simulink model "NDT_Localization"  (R2022a)
settings: Solver=FixedStepAuto  StartTime=0.0  StopTime=10.0  RelTol=1e-3
model workspace (MAT data in the model file):
  SL_ROS_VariableLengthArrays_MaxSizes : object (value not decoded)
undefined symbols (not defined in the file or in its folder): null
libraries: ros2lib x9, robotlib x8, simulink x1
(part 4 of 12)

== system NDT_Localization/observation_callback/check_localizer/If Action Subsystem/register_measurement_impl/If Action Subsystem/If Action Subsystem/solve/angle_params/If Action Subsystem3 ==
  y : Inport
  Action Port : ActionPort  ActionPortLabel=else
  Trigonometric Function : Trigonometry  Operator=cos
  Trigonometric Function1 : Trigonometry
  Out1 : Outport
  Out2 : Outport  Port=2
  wires:
  Trigonometric Function/1 -> Out1/1
  Trigonometric Function1/1 -> Out2/1
  y/1 -> Trigonometric Function1/1, Trigonometric Function/1

== system NDT_Localization/observation_callback/check_localizer/If Action Subsystem/register_measurement_impl/If Action Subsystem/If Action Subsystem/solve/angle_params/If Action Subsystem4 ==
  Action Port : ActionPort  ActionPortLabel=if(u1 > u2)
  Constant : Constant
  Constant1 : Constant  Value=0
  Out1 : Outport
  Out2 : Outport  Port=2
  wires:
  Constant/1 -> Out1/1
  Constant1/1 -> Out2/1

== system NDT_Localization/observation_callback/check_localizer/If Action Subsystem/register_measurement_impl/If Action Subsystem/If Action Subsystem/solve/angle_params/If Action Subsystem5 ==
  z : Inport
  Action Port : ActionPort  ActionPortLabel=else
  Trigonometric Function : Trigonometry  Operator=cos
  Trigonometric Function1 : Trigonometry
  Out1 : Outport
  Out2 : Outport  Port=2
  wires:
  Trigonometric Function1/1 -> Out2/1
  Trigonometric Function/1 -> Out1/1
  z/1 -> Trigonometric Function1/1, Trigonometric Function/1

== system NDT_Localization/map_callback/check_localizer/set_map/set_map_impl/insert/insert_/validate_pcl_map/check_fields/check_fields_name/For Iterator Subsystem ==
  In1 : Inport
  fields : Inport  Port=2
  ASCII to String : ASCIIToString
  Bus Selector2 : BusSelector  OutputSignals=name,offset
  Delay : Delay  DelayLength=1
  Delay1 : Delay  DelayLength=1
  For Iterator : ForIterator  IterationSource=external
  MATLAB Function : MATLAB Function  TreatAsAtomicUnit=on
  Selector : Selector  InputPortWidth=16  IndexOptions=Starting index (port)  Indices=[1 3]  OutputSizes=1
  name : Outport
  offset : Outport  Port=2
  wires:
  In1/1 -> For Iterator/1
  Selector/1 -> Bus Selector2/1  "field"
  fields/1 -> Selector/1
  Bus Selector2/1 -> ASCII to String/1  "<name>"
  Delay/1 -> MATLAB Function/1("data ")
  MATLAB Function/1(data) -> Delay/1, name/1
  For Iterator/1 -> Selector/2, MATLAB Function/2(index)  "index"
  ASCII to String/1 -> MATLAB Function/3(name)
  Bus Selector2/2 -> MATLAB Function/4(offset)  "<offset>"
  MATLAB Function/2(data1) -> Delay1/1, offset/1
  Delay1/1 -> MATLAB Function/5("data1 ")

== system NDT_Localization/map_callback/check_localizer/set_map/set_map_impl/insert/insert_/validate_pcl_map/check_fields/check_fields_name/For Iterator Subsystem1 ==
  In2 : Inport
  name : Inport  Port=2
  names : Inport  Port=3
  msg : Inport  Port=4
  Data Type Conversion : DataTypeConversion  OutDataTypeStr=uint8  SaturateOnIntegerOverflow=off  RndMeth=Floor
  Delay : Delay  DelayLength=1
  For Iterator : ForIterator  IterationSource=external
  If : If  IfExpression=u1 == 0
  If Action Subsystem : Subsystem  TreatAsAtomicUnit=on
  If Action Subsystem1 : Subsystem  TreatAsAtomicUnit=on
  Logical Operator : Logic  AllPortsSameDT=off  OutDataTypeStr=boolean
  MATLAB Function : MATLAB Function  TreatAsAtomicUnit=on
  Merge : Merge
  String Compare : StringCompare
  Out1 : Outport
  ret : Outport  Port=2
  wires:
  name/1 -> MATLAB Function/2(name)
  In2/1 -> For Iterator/1
  For Iterator/1 -> MATLAB Function/1(index)
  names/1 -> MATLAB Function/3(data)
  MATLAB Function/1(name_o) -> String Compare/1
  MATLAB Function/2(fields) -> String Compare/2
  String Compare/1 -> Logical Operator/2
  Logical Operator/1 -> Data Type Conversion/1, Delay/1
  Delay/1 -> Logical Operator/1
  Data Type Conversion/1 -> If/1
  If Action Subsystem/1(Out1) -> Merge/1
  If/1 -> If Action Subsystem/Action
  If/2 -> If Action Subsystem1/Action
  If Action Subsystem1/1(Out1) -> Merge/2
  msg/1 -> If Action Subsystem1/1(msg)
  Merge/1 -> Out1/1
  If Action Subsystem1/2(ret) -> ret/1

== system NDT_Localization/observation_callback/check_localizer/If Action Subsystem/register_measurement_impl/If Action Subsystem/If Action Subsystem/solve/If Action Subsystem1/For Iterator Subsystem/For Iterator Subsystem ==
  data : Inport
  myu : Inport  Port=2
  sigma : Inport  Port=3
  outlier_ratio : Inport  Port=4
  voxel_size_x : Inport  Port=5
  voxel_size_y : Inport  Port=6
  voxel_size_z : Inport  Port=7
  set_jacobian : Inport  Port=8
  set_gradient : Inport  Port=9
  set_hessian : Inport  Port=10
  point_hessian : Inport  Port=11
  Affine : MATLAB Function  TreatAsAtomicUnit=on
  Delay : Delay  DelayLength=1
  For Iterator : ForIterator  IterationSource=external
  For Iterator Subsystem : Subsystem  TreatAsAtomicUnit=on
  MATLAB Function : MATLAB Function  TreatAsAtomicUnit=on
  Width : Width
  gradient_jaco : Subsystem
  make_c_param : Subsystem
  make_d_param : Subsystem
  score : Subsystem
  score_out : Outport
  jacobian_out : Outport  Port=2
  hessian_out : Outport  Port=3
  wires:
  make_c_param/1(c1) -> make_d_param/1(c1)
  voxel_size_z/1 -> make_c_param/4(voxel_size_z)
  outlier_ratio/1 -> make_c_param/1(outlier_ratio)
  make_d_param/2(d2) -> For Iterator Subsystem/9(d2), gradient_jaco/9(d2), score/6(d2)
  voxel_size_y/1 -> make_c_param/3(voxel_size_y)
  make_c_param/2(c2) -> make_d_param/2(c2)
  voxel_size_x/1 -> make_c_param/2(voxel_size_x)
  make_d_param/1(d1) -> For Iterator Subsystem/8(d1), score/5(d1), gradient_jaco/8(d1)
  Width/1 -> For Iterator/1
  For Iterator/1 -> For Iterator Subsystem/3(i), gradient_jaco/3(index), MATLAB Function/2(index)
  MATLAB Function/1(pt) -> Affine/1(u)
  Affine/1(out) -> score/4(x), For Iterator Subsystem/4(data), gradient_jaco/4(data)
  sigma/1 -> For Iterator Subsystem/5(sigma), score/2(sigma), gradient_jaco/5(sigma)
  myu/1 -> gradient_jaco/6(myu), For Iterator Subsystem/6(myu), score/3(myu)
  score/1(p) -> score_out/1, Delay/1
  Delay/1 -> score/1(score)
  set_jacobian/1 -> gradient_jaco/1(set_jacobian)
  gradient_jaco/1(Out1) -> jacobian_out/1
  set_gradient/1 -> For Iterator Subsystem/2(set_gradient), gradient_jaco/2(set_gradient)
  set_hessian/1 -> For Iterator Subsystem/1(set_hessian)
  data/1 -> For Iterator Subsystem/7(x), gradient_jaco/7(x), MATLAB Function/1(data), Width/1
  point_hessian/1 -> For Iterator Subsystem/10(point_hessian)
  For Iterator Subsystem/1(Out1) -> hessian_out/1

== system NDT_Localization/observation_callback/check_localizer/If Action Subsystem/register_measurement_impl/If Action Subsystem/If Action Subsystem/solve/If Action Subsystem1/For Iterator Subsystem/If Action Subsystem ==
  opt_direction.norm : Inport
  nr_iterations : Inport  Port=2
  Action Port : ActionPort  ActionPortLabel=if(u1 == 0 & u2 == 0 & u3 == 0 & u4 == 0)
  Bus Creator : BusCreator  Inputs=3
  termination_type.FAILURE : Constant  Value=2  OutDataTypeStr=uint32
  Out1 : Outport
  wires:
  Bus Creator/1 -> Out1/1  "OptimizationSummary"
  termination_type.FAILURE/1 -> Bus Creator/2  "termination_type"
  nr_iterations/1 -> Bus Creator/3
  opt_direction.norm/1 -> Bus Creator/1

== system NDT_Localization/observation_callback/check_localizer/If Action Subsystem/register_measurement_impl/If Action Subsystem/If Action Subsystem/solve/If Action Subsystem1/For Iterator Subsystem/If Action Subsystem1 ==
  opt_direction.norm : Inport
  nr_iterations : Inport  Port=2
  Action Port : ActionPort  ActionPortLabel=elseif(u5 <= u6)
  Bus Creator : BusCreator  Inputs=3
  termination_type.CONVERGENCE : Constant  OutDataTypeStr=uint32
  Out1 : Outport
  wires:
  termination_type.CONVERGENCE/1 -> Bus Creator/2  "termination_type"
  Bus Creator/1 -> Out1/1  "OptimizationSummary"
  nr_iterations/1 -> Bus Creator/3
  opt_direction.norm/1 -> Bus Creator/1

== system NDT_Localization/observation_callback/check_localizer/If Action Subsystem/register_measurement_impl/If Action Subsystem/If Action Subsystem/solve/If Action Subsystem1/For Iterator Subsystem/If Action Subsystem2 ==
  opt_direction.norm : Inport
  nr_iterations : Inport  Port=2
  Action Port : ActionPort  ActionPortLabel=else
  Bus Creator : BusCreator  Inputs=3
  termination_type.FAILURE : Constant  Value=2  OutDataTypeStr=uint32
  Out1 : Outport
  wires:
  termination_type.FAILURE/1 -> Bus Creator/2  "termination_type"
  Bus Creator/1 -> Out1/1  "OptimizationSummary"
  nr_iterations/1 -> Bus Creator/3
  opt_direction.norm/1 -> Bus Creator/1

== system NDT_Localization/observation_callback/check_localizer/If Action Subsystem/register_measurement_impl/If Action Subsystem/If Action Subsystem/solve/If Action Subsystem1/For Iterator Subsystem/angle_params ==
  pose : Inport
  Bus Creator : BusCreator  Inputs=6
  If : If  NumInputs=2  IfExpression=u1 > u2
  If Action Subsystem : Subsystem  TreatAsAtomicUnit=on
  If Action Subsystem1 : Subsystem  TreatAsAtomicUnit=on
  If Action Subsystem2 : Subsystem  TreatAsAtomicUnit=on
  If Action Subsystem3 : Subsystem  TreatAsAtomicUnit=on
  If Action Subsystem4 : Subsystem  TreatAsAtomicUnit=on
  If Action Subsystem5 : Subsystem  TreatAsAtomicUnit=on
  If1 : If  NumInputs=2  IfExpression=u1 > u2
  If2 : If  NumInputs=2  IfExpression=u1 > u2
  MATLAB Function : MATLAB Function  TreatAsAtomicUnit=on
  Merge{,1..5} (6 alike) : Merge
  approx_thresh : Constant  Value=0.00010
  params : Outport
  wires:
  pose/1 -> MATLAB Function/1(u)
  MATLAB Function/1(x) -> If/2, If Action Subsystem1/1(x)
  MATLAB Function/3(z) -> If2/2, If Action Subsystem5/1(z)
  MATLAB Function/2(y) -> If Action Subsystem3/1(y), If1/2
  If Action Subsystem1/1(Out1) -> Merge/2
  If Action Subsystem1/2(Out2) -> Merge1/2
  If Action Subsystem3/1(Out1) -> Merge2/2
  If Action Subsystem3/2(Out2) -> Merge3/2
  If Action Subsystem5/1(Out1) -> Merge4/2
  If Action Subsystem5/2(Out2) -> Merge5/2
  approx_thresh/1 -> If2/1, If1/1, If/1
  If/1 -> If Action Subsystem/Action
  If/2 -> If Action Subsystem1/Action
  If1/1 -> If Action Subsystem2/Action
  If1/2 -> If Action Subsystem3/Action
  If2/2 -> If Action Subsystem5/Action
  If2/1 -> If Action Subsystem4/Action
  If Action Subsystem/1(Out1) -> Merge/1
  If Action Subsystem/2(Out2) -> Merge1/1
  If Action Subsystem2/1(Out1) -> Merge2/1
  If Action Subsystem2/2(Out2) -> Merge3/1
  If Action Subsystem4/1(Out1) -> Merge4/1
  If Action Subsystem4/2(Out2) -> Merge5/1
  Bus Creator/1 -> params/1
  Merge/1 -> Bus Creator/1  "cx"
  Merge1/1 -> Bus Creator/2  "sx"
  Merge2/1 -> Bus Creator/3  "cy"
  Merge3/1 -> Bus Creator/4  "sy"
  Merge4/1 -> Bus Creator/5  "cz"
  Merge5/1 -> Bus Creator/6  "sz"

== system NDT_Localization/observation_callback/check_localizer/If Action Subsystem/register_measurement_impl/If Action Subsystem/If Action Subsystem/solve/If Action Subsystem1/For Iterator Subsystem/compute_next_step ==
  eig_pose : Inport
  opt_direction : Inport  Port=2
  problem : Inport  Port=3
  localizer_ptr : Inport  Port=4
  Add4 : Sum  Inputs=+
  Bus Selector : BusSelector  OutputSignals=OptimizerT.MoreThuenteLineSearch.max_step,OptimizerT.MoreThuenteLineSearch.min_step
  If : If  NumInputs=2  IfExpression=u1 < u2
  If Action Subsystem : Subsystem  TreatAsAtomicUnit=on
  If Action Subsystem1 : Subsystem  TreatAsAtomicUnit=on
  Math Function2 : Math  Operator=square
  Merge : Merge
  Min : MinMax  Inputs=2
  step : Outport
  wires:
  Merge/1 -> step/1
  Math Function2/1 -> Add4/1
  opt_direction/1 -> If Action Subsystem1/3(opt_direction), If Action Subsystem/1(opt_direction), Math Function2/1
  localizer_ptr/1 -> If Action Subsystem1/5(localizer_ptr), Bus Selector/1
  Bus Selector/2 -> If/2  "<min_step>"
  Add4/1 -> Min/1  "step_norm"
  Bus Selector/1 -> Min/2  "<max_step>"
  Min/1 -> If Action Subsystem1/1(a_t), If/1  "a_t"
  If/2 -> If Action Subsystem1/Action
  If/1 -> If Action Subsystem/Action
  If Action Subsystem/1(Out1) -> Merge/1
  If Action Subsystem1/1(Out1) -> Merge/2
  eig_pose/1 -> If Action Subsystem1/2(eig_pose)
  problem/1 -> If Action Subsystem1/4(problem)

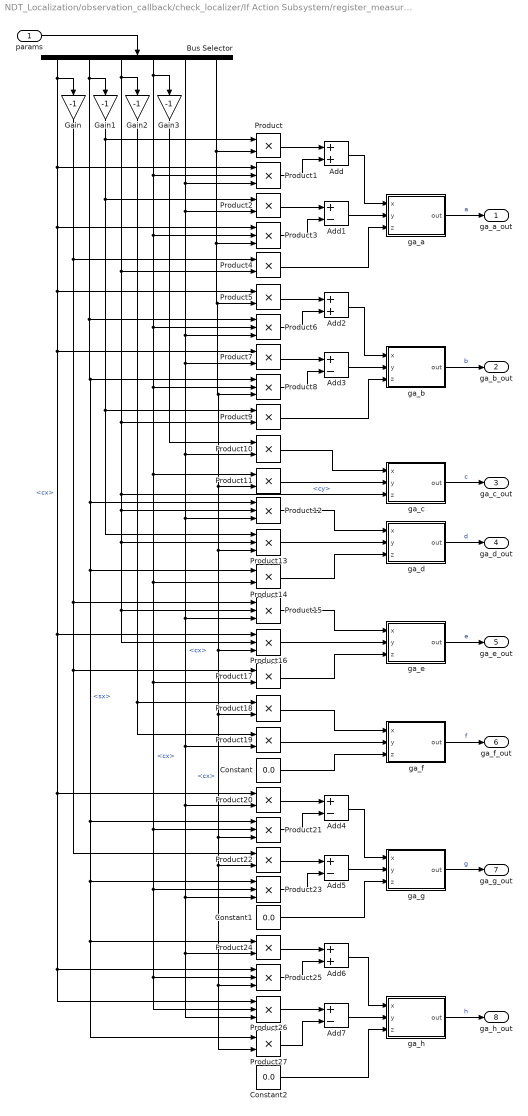
== system NDT_Localization/observation_callback/check_localizer/If Action Subsystem/register_measurement_impl/If Action Subsystem/If Action Subsystem/solve/If Action Subsystem1/For Iterator Subsystem/gradient_angle ==
  params : Inport
  Add : Sum
  Add{1,3..5,7} (5 alike) : Sum  Inputs=+-
  Add2 : Sum
  Add6 : Sum
  Bus Selector : BusSelector  OutputSignals=cx,sx,cy,sy,cz,sz
  Constant : Constant  Value=0.0
  Constant1 : Constant  Value=0.0
  Constant2 : Constant  Value=0.0
  Gain{,1..3} (4 alike) : Gain  Gain=-1
  Product{,2,4..5,7,9..11,14,17..20,22,24,27} (16 alike) : Product
  Product{1,3,6,8,12..13,15..16,21,23,25..26} (12 alike) : Product  Inputs=3
  ga_a : MATLAB Function  TreatAsAtomicUnit=on
  ga_b : MATLAB Function  TreatAsAtomicUnit=on
  ga_c : MATLAB Function  TreatAsAtomicUnit=on
  ga_d : MATLAB Function  TreatAsAtomicUnit=on
  ga_e : MATLAB Function  TreatAsAtomicUnit=on
  ga_f : MATLAB Function  TreatAsAtomicUnit=on
  ga_g : MATLAB Function  TreatAsAtomicUnit=on
  ga_h : MATLAB Function  TreatAsAtomicUnit=on
  ga_a_out : Outport
  ga_b_out : Outport  Port=2
  ga_c_out : Outport  Port=3
  ga_d_out : Outport  Port=4
  ga_e_out : Outport  Port=5
  ga_f_out : Outport  Port=6
  ga_g_out : Outport  Port=7
  ga_h_out : Outport  Port=8
  wires:
  params/1 -> Bus Selector/1
  Bus Selector/1 -> Product1/1, Product16/1, Product25/1, Product26/1, Product20/1, Product7/1, Product5/1, Product3/1, Gain/1  "<cx>"
  Bus Selector/2 -> Product6/1, Product12/1, Product14/1, Product21/1, Product23/1, Product27/1, Product24/1, Product8/1, Gain1/1  "<sx>"
  Bus Selector/3 -> Product12/2, Product13/2, Product15/2, Product16/2, ga_c/3(z), Product9/2, Product4/2, Gain2/1  "<cy>"
  Bus Selector/4 -> Product11/1, Product14/2, Product17/2, Product21/2, Product25/2, Product26/2, Product23/2, Product8/2, Product6/2, Product3/2, Product1/2, Gain3/1  "<cx>"
  Bus Selector/5 -> Product6/3, Product10/2, Product12/3, Product15/3, Product19/2, Product20/2, Product23/3, Product26/3, Product24/2, Product7/2, Product2/2, Product1/3  "<cx>"
  Bus Selector/6 -> Product11/2, Product13/3, Product16/3, Product18/2, Product21/3, Product22/2, Product25/3, Product27/2, Product8/3, Product5/2, Product3/3, Product/2  "<cx>"
  Gain1/1 -> Product13/1, Product9/1, Product2/1, Product/1
  Product/1 -> Add/1
  Product1/1 -> Add/2
  Product2/1 -> Add1/1
  Add/1 -> ga_a/1(x)
  Add1/1 -> ga_a/2(y)
  Gain/1 -> Product15/1, Product17/1, Product22/1, Product4/1
  Product4/1 -> ga_a/3(z)
  Product3/1 -> Add1/2
  Product6/1 -> Add2/2
  Product7/1 -> Add3/1
  Product8/1 -> Add3/2
  Product5/1 -> Add2/1
  Add2/1 -> ga_b/1(x)
  Product9/1 -> ga_b/3(z)
  Add3/1 -> ga_b/2(y)
  Product11/1 -> ga_c/2(y)
  Product10/1 -> ga_c/1(x)
  Gain2/1 -> Product18/1, Product19/1
  Gain3/1 -> Product10/1
  Product13/1 -> ga_d/2(y)
  Product12/1 -> ga_d/1(x)
  Product14/1 -> ga_d/3(z)
  Product19/1 -> ga_f/2(y)
  Constant/1 -> ga_f/3(z)
  Product18/1 -> ga_f/1(x)
  Product16/1 -> ga_e/2(y)
  Product17/1 -> ga_e/3(z)
  Product15/1 -> ga_e/1(x)
  Product21/1 -> Add4/2
  Product22/1 -> Add5/1
  Product23/1 -> Add5/2
  Product20/1 -> Add4/1
  Add5/1 -> ga_g/2(y)
  Product25/1 -> Add6/2
  Product26/1 -> Add7/1
  Product27/1 -> Add7/2
  Product24/1 -> Add6/1
  Constant1/1 -> ga_g/3(z)
  Add4/1 -> ga_g/1(x)
  Add7/1 -> ga_h/2(y)
  Add6/1 -> ga_h/1(x)
  Constant2/1 -> ga_h/3(z)
  ga_a/1(out) -> ga_a_out/1  "a"
  ga_b/1(out) -> ga_b_out/1  "b"
  ga_c/1(out) -> ga_c_out/1  "c"
  ga_d/1(out) -> ga_d_out/1  "d"
  ga_e/1(out) -> ga_e_out/1  "e"
  ga_f/1(out) -> ga_f_out/1  "f"
  ga_g/1(out) -> ga_g_out/1  "g"
  ga_h/1(out) -> ga_h_out/1  "h"

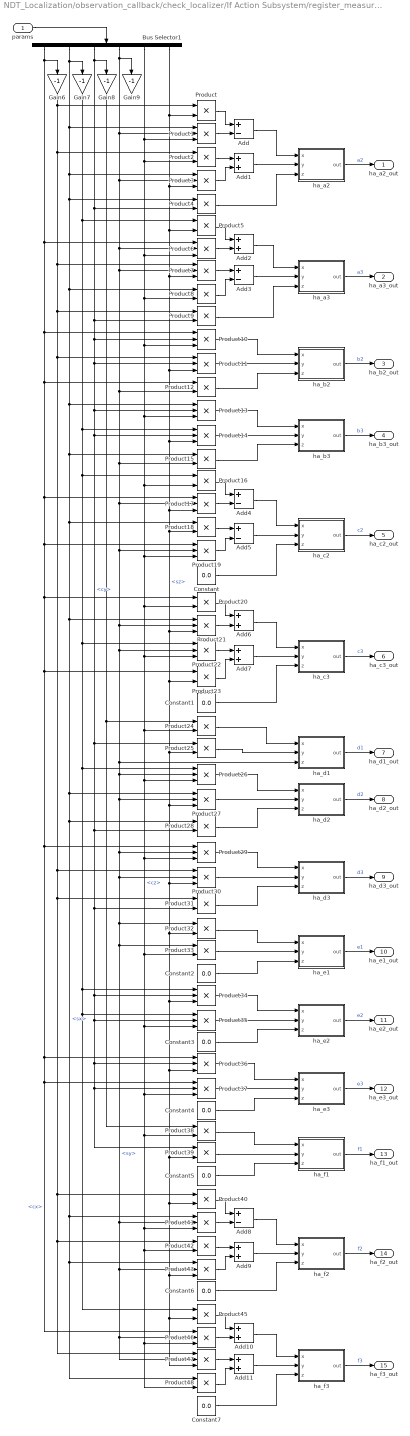
== system NDT_Localization/observation_callback/check_localizer/If Action Subsystem/register_measurement_impl/If Action Subsystem/If Action Subsystem/solve/If Action Subsystem1/For Iterator Subsystem/hessian_angle ==
  params : Inport
  Add{,3..5,8} (5 alike) : Sum  Inputs=+-
  Add{1..2,6..7,9..11} (7 alike) : Sum
  Bus Selector1 : BusSelector  OutputSignals=cx,sx,cy,sy,cz,sz
  Constant{,1..7} (8 alike) : Constant  Value=0.0
  Gain{6..9} (4 alike) : Gain  Gain=-1
  Product{,2,4..5,8..9,12,15..16,18,20,23..25,28,31..33,38..40,42,45,48} (24 alike) : Product
  Product{1,3,6..7,10..11,13..14,17,19,21..22,26..27,29..30,34..37,41,43,46..47} (24 alike) : Product  Inputs=3
  ha_a2 : MATLAB Function  TreatAsAtomicUnit=on
  ha_a3 : MATLAB Function  TreatAsAtomicUnit=on
  ha_b2 : MATLAB Function  TreatAsAtomicUnit=on
  ha_b3 : MATLAB Function  TreatAsAtomicUnit=on
  ha_c2 : MATLAB Function  TreatAsAtomicUnit=on
  ha_c3 : MATLAB Function  TreatAsAtomicUnit=on
  ha_d1 : MATLAB Function  TreatAsAtomicUnit=on
  ha_d2 : MATLAB Function  TreatAsAtomicUnit=on
  ha_d3 : MATLAB Function  TreatAsAtomicUnit=on
  ha_e1 : MATLAB Function  TreatAsAtomicUnit=on
  ha_e2 : MATLAB Function  TreatAsAtomicUnit=on
  ha_e3 : MATLAB Function  TreatAsAtomicUnit=on
  ha_f1 : MATLAB Function  TreatAsAtomicUnit=on
  ha_f2 : MATLAB Function  TreatAsAtomicUnit=on
  ha_f3 : MATLAB Function  TreatAsAtomicUnit=on
  ha_a2_out : Outport
  ha_a3_out : Outport  Port=2
  ha_b2_out : Outport  Port=3
  ha_b3_out : Outport  Port=4
  ha_c2_out : Outport  Port=5
  ha_c3_out : Outport  Port=6
  ha_d1_out : Outport  Port=7
  ha_d2_out : Outport  Port=8
  ha_d3_out : Outport  Port=9
  ha_e1_out : Outport  Port=10
  ha_e2_out : Outport  Port=11
  ha_e3_out : Outport  Port=12
  ha_f1_out : Outport  Port=13
  ha_f2_out : Outport  Port=14
  ha_f3_out : Outport  Port=15
  wires:
  Bus Selector1/1 -> Product6/1, Product10/1, Product12/1, Product17/1, Product19/1, Product20/1, Product23/1, Product29/1, Product36/1, Product37/1, Product46/1, Gain6/1  "<cx>"
  Bus Selector1/3 -> Product4/2, Product9/2, Product10/2, Product11/2, Product13/2, Product14/2, Product25/1, Product28/2, Product31/2, Product34/2, Product35/2, Product36/2, Product37/2, Product39/1, Gain8/1  "<cy>"
  Bus Selector1/4 -> Product1/2, Product3/2, Product6/2, Product7/2, Product15/2, Product17/2, Product19/2, ha_d1/3(z), Product27/2, Product29/2, Product30/2, Product32/1, Product33/1, Product41/2, Product43/2, Product47/2, Product46/2, Product26/2, Product22/2, Product21/2, Product12/2, Gain9/1  "<sy>"
  params/1 -> Bus Selector1/1
  Bus Selector1/2 -> Product1/1, Product3/1, Product4/1, Product8/1, Product13/1, Product15/1, Product18/1, Product21/1, Product27/1, Product28/1, Product41/1, Product43/1, Product48/1, Gain7/1  "<sx>"
  Bus Selector1/5 -> Product1/3, Product2/2, Product6/3, Product8/2, Product10/3, Product13/3, Product16/2, Product19/3, Product20/2, Product22/3, Product24/2, Product26/3, Product29/3, Product33/2, Product35/3, Product37/3, Product38/2, Product41/3, Product42/2, Product46/3, Product48/2  "<cz>"
  Bus Selector1/6 -> Product/2, Product3/3, Product5/2, Product7/3, Product11/3, Product14/3, Product17/3, Product18/2, Product21/3, Product23/2, Product25/2, Product30/3, Product32/2, Product34/3, Product36/3, Product39/2, Product40/2, Product43/3, Product45/2, Product47/3, Product27/3  "<sz>"
  ha_a2/1(out) -> ha_a2_out/1  "a2"
  ha_a3/1(out) -> ha_a3_out/1  "a3"
  ha_b3/1(out) -> ha_b3_out/1  "b3"
  ha_b2/1(out) -> ha_b2_out/1  "b2"
  ha_c3/1(out) -> ha_c3_out/1  "c3"
  ha_c2/1(out) -> ha_c2_out/1  "c2"
  ha_d3/1(out) -> ha_d3_out/1  "d3"
  ha_d2/1(out) -> ha_d2_out/1  "d2"
  ha_d1/1(out) -> ha_d1_out/1  "d1"
  ha_e1/1(out) -> ha_e1_out/1  "e1"
  ha_e3/1(out) -> ha_e3_out/1  "e3"
  ha_e2/1(out) -> ha_e2_out/1  "e2"
  ha_f1/1(out) -> ha_f1_out/1  "f1"
  ha_f3/1(out) -> ha_f3_out/1  "f3"
  ha_f2/1(out) -> ha_f2_out/1  "f2"
  Product1/1 -> Add/2
  Product/1 -> Add/1
  Product2/1 -> Add1/1
  Product3/1 -> Add1/2
  Product4/1 -> ha_a2/3(z)
  Add1/1 -> ha_a2/2(y)
  Add/1 -> ha_a2/1(x)
  Product9/1 -> ha_a3/3(z)
  Add3/1 -> ha_a3/2(y)
  Product8/1 -> Add3/2
  Product7/1 -> Add3/1
  Product6/1 -> Add2/2
  Product5/1 -> Add2/1
  Add2/1 -> ha_a3/1(x)
  Product11/1 -> ha_b2/2(y)
  Product10/1 -> ha_b2/1(x)
  Product12/1 -> ha_b2/3(z)
  Product14/1 -> ha_b3/2(y)
  Product13/1 -> ha_b3/1(x)
  Product15/1 -> ha_b3/3(z)
  Product19/1 -> Add5/2
  Product18/1 -> Add5/1
  Product17/1 -> Add4/2
  Product16/1 -> Add4/1
  Product23/1 -> Add7/2
  Product22/1 -> Add7/1
  Product21/1 -> Add6/2
  Product20/1 -> Add6/1
  Add5/1 -> ha_c2/2(y)
  Constant/1 -> ha_c2/3(z)
  Add4/1 -> ha_c2/1(x)
  Add7/1 -> ha_c3/2(y)
  Constant1/1 -> ha_c3/3(z)
  Add6/1 -> ha_c3/1(x)
  Product25/1 -> ha_d1/2(y)
  Product24/1 -> ha_d1/1(x)
  Product27/1 -> ha_d2/2(y)
  Product28/1 -> ha_d2/3(z)
  Product26/1 -> ha_d2/1(x)
  Product30/1 -> ha_d3/2(y)
  Product29/1 -> ha_d3/1(x)
  Product31/1 -> ha_d3/3(z)
  Product33/1 -> ha_e1/2(y)
  Product32/1 -> ha_e1/1(x)
  Constant2/1 -> ha_e1/3(z)
  Product35/1 -> ha_e2/2(y)
  Product34/1 -> ha_e2/1(x)
  Constant3/1 -> ha_e2/3(z)
  Constant4/1 -> ha_e3/3(z)
  Product37/1 -> ha_e3/2(y)
  Product36/1 -> ha_e3/1(x)
  Constant5/1 -> ha_f1/3(z)
  Product38/1 -> ha_f1/1(x)
  Product39/1 -> ha_f1/2(y)
  Product42/1 -> Add9/1
  Product41/1 -> Add8/2
  Product46/1 -> Add10/2
  Product48/1 -> Add11/2
  Product43/1 -> Add9/2
  Product40/1 -> Add8/1
  Product47/1 -> Add11/1
  Product45/1 -> Add10/1
  Add9/1 -> ha_f2/2(y)
  Add11/1 -> ha_f3/2(y)
  Add10/1 -> ha_f3/1(x)
  Add8/1 -> ha_f2/1(x)
  Constant6/1 -> ha_f2/3(z)
  Constant7/1 -> ha_f3/3(z)
  Gain7/1 -> Product5/1, Product14/1, Product16/1, Product22/1, Product34/1, Product35/1, Product45/1, Product26/1
  Gain8/1 -> Product24/1, Product38/1
  Gain6/1 -> Product2/1, Product7/1, Product9/1, Product11/1, Product30/1, Product31/1, Product40/1, Product42/1, Product47/1, Product/1

== system NDT_Localization/map_callback/check_localizer/set_map/set_map_impl/insert/insert_/validate_pcl_map/check_fields/check_fields_name/For Iterator Subsystem1/If Action Subsystem ==
  Action Port : ActionPort  ActionPortLabel=if(u1 == 0)
  Constant : Constant  Value=0
  Out1 : Outport
  wires:
  Constant/1 -> Out1/1

== system NDT_Localization/map_callback/check_localizer/set_map/set_map_impl/insert/insert_/validate_pcl_map/check_fields/check_fields_name/For Iterator Subsystem1/If Action Subsystem1 ==
  msg : Inport
  Action Port : ActionPort  ActionPortLabel=else
  Add : Sum  Inputs=+-
  Bus Selector : BusSelector  OutputSignals=data,row_step,width,point_step
  Constant : Constant
  Divide : Product  Inputs=*/
  Math Function : Math  Operator=mod
  Min : MinMax  Inputs=3
  Product : Product
  Width : Width
  Out1 : Outport
  ret : Outport  Port=2
  wires:
  msg/1 -> Bus Selector/1
  Constant/1 -> Out1/1
  Bus Selector/1 -> Width/1  "<data>"
  Width/1 -> Min/1
  Product/1 -> Min/3
  Bus Selector/4 -> Math Function/2, Divide/2, Product/2  "<point_step>"
  Bus Selector/2 -> Min/2  "<row_step>"
  Bus Selector/3 -> Product/1  "<width>"
  Min/1 -> Add/1, Math Function/1  "min_data_length"
  Math Function/1 -> Add/2
  Add/1 -> Divide/1  "safe_data_length"
  Divide/1 -> ret/1

== system NDT_Localization/observation_callback/check_localizer/If Action Subsystem/register_measurement_impl/If Action Subsystem/If Action Subsystem/solve/If Action Subsystem1/For Iterator Subsystem/For Iterator Subsystem/For Iterator Subsystem ==
  set_hessian : Inport
  set_gradient : Inport  Port=2
  i : Inport  Port=3
  data : Inport  Port=4
  sigma : Inport  Port=5
  myu : Inport  Port=6
  x : Inport  Port=7
  d1 : Inport  Port=8
  d2 : Inport  Port=9
  point_hessian : Inport  Port=10
  Add : Sum  Inputs=+-
  Add1 : Sum  Inputs=+++
  Constant : Constant  Value=-2
  Divide1 : Product  Inputs=*/
  For Iterator : ForIterator  IterationSource=external
  MATLAB Function : MATLAB Function  TreatAsAtomicUnit=on
  MATLAB Function1 : MATLAB Function  TreatAsAtomicUnit=on
  Math Function : Math
  Math Function1 : Math  Operator=transpose
  Math Function2 : Math  Operator=reciprocal
  Product : Product  Inputs=4
  Product1 : Product  Inputs=3  Multiplication=Matrix(*)
  Product{4,6,8,10} (4 alike) : Product  Multiplication=Matrix(*)
  Product{2..3,5,7,9} (5 alike) : Product
  gradient_col_i : MATLAB Function  TreatAsAtomicUnit=on
  gradient_col_j : MATLAB Function  TreatAsAtomicUnit=on
  hessian_add : MATLAB Function  TreatAsAtomicUnit=on
  Out1 : Outport
  wires:
  Product3/1 -> Product8/2, Product4/2
  Product4/1 -> Product7/1
  Constant/1 -> Divide1/2
  set_gradient/1 -> gradient_col_j/2(gradient), gradient_col_i/2(gradient)
  hessian_add/1(hessian) -> Out1/1
  set_hessian/1 -> MATLAB Function/1(u), hessian_add/1("hessian ")
  i/1 -> hessian_add/2(index_i), gradient_col_i/1(index_i), MATLAB Function1/1(index_i)
  sigma/1 -> Math Function2/1
  Product/1 -> hessian_add/4(num)
  gradient_col_i/1(y) -> Product3/2
  data/1 -> Product10/1, Product6/1, Product4/1
  Add/1 -> Product1/3, Math Function1/1  "x-myu"
  d2/1 -> Divide1/1, Product/3  "d2"
  Product2/1 -> Math Function/1
  Divide1/1 -> Product2/1
  Math Function/1 -> Product/4
  Math Function1/1 -> Product1/1
  x/1 -> Add/1
  d1/1 -> Product/2  "d1"
  Product1/1 -> Product2/2
  myu/1 -> Add/2
  Math Function2/1 -> Product5/1, Product3/1, Product9/1, Product1/2  "inv_cov"
  MATLAB Function/1(y) -> For Iterator/1
  For Iterator/1 -> hessian_add/3(index_j), MATLAB Function1/2(index_j), gradient_col_j/1(index_j)
  Product5/1 -> Product6/2
  gradient_col_j/1(y) -> Product8/1, Product5/2
  Product6/1 -> Product7/2
  Product7/1 -> Add1/1
  Add1/1 -> Product/1
  Product8/1 -> Add1/3
  Product9/1 -> Product10/2
  Product10/1 -> Add1/2
  point_hessian/1 -> MATLAB Function1/3(point_hessian)
  MATLAB Function1/1(y) -> Product9/2

== system NDT_Localization/observation_callback/check_localizer/If Action Subsystem/register_measurement_impl/If Action Subsystem/If Action Subsystem/solve/If Action Subsystem1/For Iterator Subsystem/For Iterator Subsystem/gradient_jaco ==
  set_jacobian : Inport
  set_gradient : Inport  Port=2
  index : Inport  Port=3
  data : Inport  Port=4
  sigma : Inport  Port=5
  myu : Inport  Port=6
  x : Inport  Port=7
  d1 : Inport  Port=8
  d2 : Inport  Port=9
  Add : Sum  Inputs=+-
  Constant : Constant  Value=-2
  Divide1 : Product  Inputs=*/
  Math Function : Math
  Math Function1 : Math  Operator=transpose
  Math Function2 : Math  Operator=reciprocal
  Product : Product  Inputs=4
  Product1 : Product  Inputs=3  Multiplication=Matrix(*)
  Product2 : Product
  Product3 : Product
  Product4 : Product  Multiplication=Matrix(*)
  gradient_col : MATLAB Function  TreatAsAtomicUnit=on
  jaco_add : MATLAB Function  TreatAsAtomicUnit=on
  Out1 : Outport
  wires:
  myu/1 -> Add/2
  Constant/1 -> Divide1/2
  Math Function1/1 -> Product1/1
  Divide1/1 -> Product2/1
  d2/1 -> Divide1/1, Product/3  "d2"
  Math Function2/1 -> Product3/2, Product1/2  "inv_cov"
  Product1/1 -> Product2/2
  d1/1 -> Product/2  "d1"
  x/1 -> Add/1
  Math Function/1 -> Product/4
  Product2/1 -> Math Function/1
  Add/1 -> Product1/3, Math Function1/1  "x-myu"
  sigma/1 -> Math Function2/1
  Product/1 -> jaco_add/3(num)
  index/1 -> jaco_add/2(index), gradient_col/1(index)
  jaco_add/1(jacobian) -> Out1/1
  set_jacobian/1 -> jaco_add/1("jacobian ")
  set_gradient/1 -> gradient_col/2(gradient)
  gradient_col/1(y) -> Product3/1
  data/1 -> Product4/1
  Product3/1 -> Product4/2
  Product4/1 -> Product/1

== system NDT_Localization/observation_callback/check_localizer/If Action Subsystem/register_measurement_impl/If Action Subsystem/If Action Subsystem/solve/If Action Subsystem1/For Iterator Subsystem/For Iterator Subsystem/make_c_param ==
  outlier_ratio : Inport
  voxel_size_x : Inport  Port=2
  voxel_size_y : Inport  Port=3
  voxel_size_z : Inport  Port=4
  Constant : Constant
  Divide : Product  Inputs=*/
  Gain : Gain  Gain=10
  Product : Product  Inputs=3
  Subtract : Sum  Inputs=+-
  c1 : Outport
  c2 : Outport  Port=2
  wires:
  Constant/1 -> Subtract/1
  outlier_ratio/1 -> Divide/1, Subtract/2
  Subtract/1 -> Gain/1
  Gain/1 -> c1/1
  Product/1 -> Divide/2
  Divide/1 -> c2/1
  voxel_size_y/1 -> Product/2
  voxel_size_z/1 -> Product/3
  voxel_size_x/1 -> Product/1

== system NDT_Localization/observation_callback/check_localizer/If Action Subsystem/register_measurement_impl/If Action Subsystem/If Action Subsystem/solve/If Action Subsystem1/For Iterator Subsystem/For Iterator Subsystem/make_d_param ==
  c1 : Inport
  c2 : Inport  Port=2
  Add1 : Sum
  Add2 : Sum  Inputs=-+
  Add3 : Sum
  Add4 : Sum  Inputs=+-
  Constant : Constant  Value=-2
  Constant1 : Constant  Value=-0.5
  Divide : Product  Inputs=*/
  Math Function{3..4,6..7} (4 alike) : Math  Operator=log
  Math Function5 : Math
  Product3 : Product
  Product4 : Product
  d1 : Outport
  d2 : Outport  Port=2
  wires:
  Add2/1 -> Divide/2, d1/1  "d1"
  Math Function4/1 -> Add4/1, Add2/2  "-d3"
  Product4/1 -> Add3/1
  Add3/1 -> Math Function6/1
  c1/1 -> Product4/1, Add1/1
  Constant/1 -> Product3/2
  Constant1/1 -> Math Function5/1
  Product3/1 -> d2/1  "d2"
  Math Function5/1 -> Product4/2
  Math Function7/1 -> Product3/1
  Divide/1 -> Math Function7/1
  Math Function6/1 -> Add4/2
  c2/1 -> Add3/2, Math Function4/1, Add1/2
  Add4/1 -> Divide/1
  Add1/1 -> Math Function3/1
  Math Function3/1 -> Add2/1

== system NDT_Localization/observation_callback/check_localizer/If Action Subsystem/register_measurement_impl/If Action Subsystem/If Action Subsystem/solve/If Action Subsystem1/For Iterator Subsystem/For Iterator Subsystem/score ==
  score : Inport
  sigma : Inport  Port=2
  myu : Inport  Port=3
  x : Inport  Port=4
  d1 : Inport  Port=5
  d2 : Inport  Port=6
  Add : Sum  Inputs=+-
  Add1 : Sum
  Constant : Constant  Value=-2
  Divide1 : Product  Inputs=*/
  Gain : Gain  Gain=-1
  Math Function : Math
  Math Function1 : Math  Operator=transpose
  Math Function2 : Math  Operator=reciprocal
  Product : Product
  Product1 : Product  Inputs=3  Multiplication=Matrix(*)
  Product2 : Product
  p : Outport
  wires:
  sigma/1 -> Math Function2/1
  Math Function/1 -> Product/2
  Gain/1 -> Product/1  "-d1"
  myu/1 -> Add/2
  x/1 -> Add/1
  Product2/1 -> Math Function/1
  Add/1 -> Product1/3, Math Function1/1  "x-myu"
  Product/1 -> Add1/2
  Math Function1/1 -> Product1/1
  Product1/1 -> Product2/2
  Math Function2/1 -> Product1/2
  Constant/1 -> Divide1/2
  Divide1/1 -> Product2/1
  d2/1 -> Divide1/1  "d2"
  d1/1 -> Gain/1
  Add1/1 -> p/1
  score/1 -> Add1/1

== system NDT_Localization/observation_callback/check_localizer/If Action Subsystem/register_measurement_impl/If Action Subsystem/If Action Subsystem/solve/If Action Subsystem1/For Iterator Subsystem/angle_params/If Action Subsystem ==
  Action Port : ActionPort
  Constant : Constant
  Constant1 : Constant  Value=0
  Out1 : Outport
  Out2 : Outport  Port=2
  wires:
  Constant/1 -> Out1/1
  Constant1/1 -> Out2/1

== system NDT_Localization/observation_callback/check_localizer/If Action Subsystem/register_measurement_impl/If Action Subsystem/If Action Subsystem/solve/If Action Subsystem1/For Iterator Subsystem/angle_params/If Action Subsystem1 ==
  x : Inport
  Action Port : ActionPort
  Trigonometric Function : Trigonometry  Operator=cos
  Trigonometric Function1 : Trigonometry
  Out1 : Outport
  Out2 : Outport  Port=2
  wires:
  x/1 -> Trigonometric Function1/1, Trigonometric Function/1
  Trigonometric Function1/1 -> Out2/1
  Trigonometric Function/1 -> Out1/1

== system NDT_Localization/observation_callback/check_localizer/If Action Subsystem/register_measurement_impl/If Action Subsystem/If Action Subsystem/solve/If Action Subsystem1/For Iterator Subsystem/angle_params/If Action Subsystem2 ==
  Action Port : ActionPort
  Constant : Constant
  Constant1 : Constant  Value=0
  Out1 : Outport
  Out2 : Outport  Port=2
  wires:
  Constant/1 -> Out1/1
  Constant1/1 -> Out2/1

== system NDT_Localization/observation_callback/check_localizer/If Action Subsystem/register_measurement_impl/If Action Subsystem/If Action Subsystem/solve/If Action Subsystem1/For Iterator Subsystem/angle_params/If Action Subsystem3 ==
  y : Inport
  Action Port : ActionPort
  Trigonometric Function : Trigonometry  Operator=cos
  Trigonometric Function1 : Trigonometry
  Out1 : Outport
  Out2 : Outport  Port=2
  wires:
  Trigonometric Function/1 -> Out1/1
  Trigonometric Function1/1 -> Out2/1
  y/1 -> Trigonometric Function1/1, Trigonometric Function/1

== system NDT_Localization/observation_callback/check_localizer/If Action Subsystem/register_measurement_impl/If Action Subsystem/If Action Subsystem/solve/If Action Subsystem1/For Iterator Subsystem/angle_params/If Action Subsystem4 ==
  Action Port : ActionPort
  Constant : Constant
  Constant1 : Constant  Value=0
  Out1 : Outport
  Out2 : Outport  Port=2
  wires:
  Constant/1 -> Out1/1
  Constant1/1 -> Out2/1

== system NDT_Localization/observation_callback/check_localizer/If Action Subsystem/register_measurement_impl/If Action Subsystem/If Action Subsystem/solve/If Action Subsystem1/For Iterator Subsystem/angle_params/If Action Subsystem5 ==
  z : Inport
  Action Port : ActionPort
  Trigonometric Function : Trigonometry  Operator=cos
  Trigonometric Function1 : Trigonometry
  Out1 : Outport
  Out2 : Outport  Port=2
  wires:
  Trigonometric Function1/1 -> Out2/1
  Trigonometric Function/1 -> Out1/1
  z/1 -> Trigonometric Function1/1, Trigonometric Function/1

== system NDT_Localization/observation_callback/check_localizer/If Action Subsystem/register_measurement_impl/If Action Subsystem/If Action Subsystem/solve/If Action Subsystem1/For Iterator Subsystem/compute_next_step/If Action Subsystem ==
  opt_direction : Inport
  Action Port : ActionPort  ActionPortLabel=if(u1 < u2)
  Out1 : Outport
  wires:
  opt_direction/1 -> Out1/1

== system NDT_Localization/observation_callback/check_localizer/If Action Subsystem/register_measurement_impl/If Action Subsystem/If Action Subsystem/solve/If Action Subsystem1/For Iterator Subsystem/compute_next_step/If Action Subsystem1 ==
  a_t : Inport
  eig_pose : Inport  Port=2
  opt_direction : Inport  Port=3
  problem : Inport  Port=4
  localizer_ptr : Inport  Port=5
  Action Port : ActionPort  ActionPortLabel=else
  Bus Creator : BusCreator  Inputs=4
  Bus Creator1 : BusCreator  Inputs=2
  Bus Creator2 : BusCreator  Inputs=2
  Bus Selector : BusSelector  OutputSignals=OptimizerT.MoreThuenteLineSearch.optimization_direction,OptimizerT.MoreThuenteLineSearch.mu,OptimizerT.MoreThuenteLineSearch.min_step,OptimizerT.MoreThuenteLineSearch.max_step,OptimizerT.MoreThuenteLineSearch.max_iterations
  Bus Selector1 : BusSelector  OutputSignals=min_step,max_step
  Constant : Constant  Value=0.0
  For Iterator Subsystem : Subsystem  TreatAsAtomicUnit=on
  If : If  NumInputs=2  IfExpression=u1 >= u2  ShowElse=off
  f_l : Subsystem
  f_u : Subsystem
  phi_0 : Subsystem
  phi_t : Subsystem  TreatAsAtomicUnit=on
  psi_t : Subsystem
  Out1 : Outport
  wires:
  Bus Selector/2 -> Bus Creator1/2  "<mu>"
  Bus Selector/1 -> Bus Creator/4  "<optimization_direction>"
  eig_pose/1 -> Bus Creator/1  "eig_pose"
  opt_direction/1 -> Bus Creator/2  "opt_direction"
  problem/1 -> Bus Creator/3  "problem"
  Bus Selector/3 -> Bus Creator2/1  "<min_step>"
  Bus Selector/4 -> Bus Creator2/2  "<max_step>"
  Bus Creator2/1 -> Bus Selector1/1  "interval"
  Bus Selector/5 -> For Iterator Subsystem/3(max_iterations)  "<max_iterations>"
  Bus Selector1/2 -> f_u/1(a_u)  "<max_step>"
  localizer_ptr/1 -> phi_0/3(localizer_ptr), For Iterator Subsystem/4(localizer_ptr), phi_t/3(localizer_ptr), psi_t/3(localizer_ptr), f_l/3(localizer_ptr), f_u/3(localizer_ptr), Bus Selector/1
  Bus Creator/1 -> For Iterator Subsystem/1(phi), phi_0/2(phi), phi_t/2(phi), Bus Creator1/1  "phi"
  If/1 -> phi_t/Action
  a_t/1 -> If/1, psi_t/1(a_t), phi_t/1(a_t)  "a_t"
  Bus Selector1/1 -> f_l/1(a_l)  "<min_step>"
  Constant/1 -> phi_0/1(step_size), If/2
  Bus Creator1/1 -> f_u/2(psi), f_l/2(psi), psi_t/2(psi), For Iterator Subsystem/2(psi)  "psi"
  phi_0/1(phi_0) -> For Iterator Subsystem/5(phi_0)
  phi_t/1(phi_t) -> For Iterator Subsystem/6(phi_t)
  psi_t/1(psi_t) -> For Iterator Subsystem/7(psi_t)
  f_l/1(f_l) -> For Iterator Subsystem/8(f_l)
  f_u/1(f_u) -> For Iterator Subsystem/9(f_u)
  For Iterator Subsystem/1(Out1) -> Out1/1

== system NDT_Localization/observation_callback/check_localizer/If Action Subsystem/register_measurement_impl/If Action Subsystem/If Action Subsystem/solve/If Action Subsystem1/For Iterator Subsystem/compute_next_step/If Action Subsystem1/For Iterator Subsystem ==
  phi : Inport
  psi : Inport  Port=2
  max_iterations : Inport  Port=3
  localizer_ptr : Inport  Port=4
  phi_0 : Inport  Port=5
  phi_t : Inport  Port=6
  psi_t : Inport  Port=7
  f_l : Inport  Port=8
  f_u : Inport  Port=9
  Abs : Abs  SaturateOnIntegerOverflow=off
  Abs1 : Abs  SaturateOnIntegerOverflow=off
  Add : Sum
  Add1 : Sum
  Bus Selector : BusSelector  OutputSignals=step_size,value,derivative
  Bus Selector1 : BusSelector  OutputSignals=step_size,value,derivative
  Bus Selector2 : BusSelector  OutputSignals=a_t,value,derivative
  Bus Selector5 : BusSelector  OutputSignals=OptimizerT.MoreThuenteLineSearch.eta
  Constant : Constant  Value=0.0
  Constant1 : Constant
  Constant2 : Constant
  Data Type Conversion : DataTypeConversion  OutDataTypeStr=uint8  SaturateOnIntegerOverflow=off  RndMeth=Floor
  Delay : Delay  DelayLength=1
  Delay1 : Delay  DelayLength=1  InitialCondition=true
  For Iterator : ForIterator  IterationSource=external  ExternalIncrement=on
  If : If  IfExpression=u1 == 0  ShowElse=off
  If Action Subsystem : Subsystem  TreatAsAtomicUnit=on
  Logical Operator : Logic  AllPortsSameDT=off  OutDataTypeStr=boolean
  Logical Operator1 : Logic  Operator=OR  AllPortsSameDT=off  OutDataTypeStr=boolean
  Product : Product
  Relational Operator : RelationalOperator  Operator=<=  OutDataTypeStr=boolean  RndMeth=Simplest  InputSameDT=off
  Relational Operator1 : RelationalOperator  OutDataTypeStr=boolean  RndMeth=Simplest  InputSameDT=off
  Switch : Switch  Criteria=u2 ~= 0  SaturateOnIntegerOverflow=off  InputSameDT=off
  Out1 : Outport
  wires:
  ? -> Out1/1
  max_iterations/1 -> Add1/1, For Iterator/1
  For Iterator/1 -> Delay/1  "step_iterations"
  phi_0/1 -> Bus Selector/1
  phi_t/1 -> If Action Subsystem/2(phi_t), Bus Selector1/1
  psi_t/1 -> If Action Subsystem/3(psi_t), Bus Selector2/1
  f_l/1 -> If Action Subsystem/6(f_l)
  f_u/1 -> If Action Subsystem/7(f_u)
  Constant/1 -> Relational Operator/2
  Bus Selector2/2 -> Relational Operator/1  "<value>"
  Bus Selector1/3 -> Abs/1  "<derivative>"
  Bus Selector/3 -> Abs1/1  "<derivative>"
  localizer_ptr/1 -> If Action Subsystem/1(localizer_ptr), Bus Selector5/1
  Bus Selector5/1 -> Product/1  "<eta>"
  Abs1/1 -> Product/2
  Product/1 -> Relational Operator1/1
  Abs/1 -> Relational Operator1/2
  Relational Operator1/1 -> Logical Operator/1
  Relational Operator/1 -> Logical Operator/2
  If/1 -> If Action Subsystem/Action
  Data Type Conversion/1 -> If/1
  Delay/1 -> Add/1
  Constant1/1 -> Add/2
  Switch/1 -> For Iterator/2
  Add/1 -> Switch/3
  Constant2/1 -> Add1/2
  Add1/1 -> Switch/1
  Logical Operator/1 -> Data Type Conversion/1, Logical Operator1/1
  Delay1/1 -> If Action Subsystem/8(aux_function)
  If Action Subsystem/2(aux_function_out) -> Delay1/1
  If Action Subsystem/3(flag) -> Logical Operator1/2
  Logical Operator1/1 -> Switch/2
  phi/1 -> If Action Subsystem/4(phi)
  psi/1 -> If Action Subsystem/5(psi)

== system NDT_Localization/observation_callback/check_localizer/If Action Subsystem/register_measurement_impl/If Action Subsystem/If Action Subsystem/solve/If Action Subsystem1/For Iterator Subsystem/compute_next_step/If Action Subsystem1/f_l ==
  a_l : Inport
  psi : Inport  Port=2
  localizer_ptr : Inport  Port=3
  Add : Sum  Inputs=+--
  Add1 : Sum  Inputs=+-
  Bus Creator : BusCreator  Inputs=3
  Bus Selector : BusSelector  OutputSignals=phi,mu
  Bus Selector1 : BusSelector  OutputSignals=value,derivative
  Bus Selector2 : BusSelector  OutputSignals=value,derivative
  Constant : Constant  Value=0.0
  If : If  NumInputs=2  IfExpression=u1 >= u2  ShowElse=off
  Product : Product  Inputs=3
  Product1 : Product
  initial_objective_function : Subsystem
  objective_function : Subsystem  TreatAsAtomicUnit=on
  f_l : Outport
  wires:
  psi/1 -> Bus Selector/1
  a_l/1 -> Bus Creator/1, objective_function/1(step_size), Product/2, If/1  "a_t"
  If/1 -> objective_function/Action
  Constant/1 -> initial_objective_function/1(step_size), If/2
  Bus Selector/1 -> initial_objective_function/2(phi), objective_function/2(phi)  "<phi>"
  localizer_ptr/1 -> initial_objective_function/3(localizer_ptr), objective_function/3(localizer_ptr)
  Product/1 -> Add/3
  Bus Selector/2 -> Product1/1, Product/1  "<mu>"
  objective_function/1(objective_function_value) -> Bus Selector1/1
  Bus Selector1/1 -> Add/1  "<value>"
  initial_objective_function/1(initial_objective_function_value) -> Bus Selector2/1
  Bus Selector2/1 -> Add/2  "<value>"
  Bus Selector2/2 -> Product1/2, Product/3  "<derivative>"
  Add/1 -> Bus Creator/2  "value"
  Bus Selector1/2 -> Add1/1  "<derivative>"
  Product1/1 -> Add1/2
  Add1/1 -> Bus Creator/3  "derivative"
  Bus Creator/1 -> f_l/1

== system NDT_Localization/observation_callback/check_localizer/If Action Subsystem/register_measurement_impl/If Action Subsystem/If Action Subsystem/solve/If Action Subsystem1/For Iterator Subsystem/compute_next_step/If Action Subsystem1/f_u ==
  a_u : Inport
  psi : Inport  Port=2
  localizer_ptr : Inport  Port=3
  Add : Sum  Inputs=+--
  Add1 : Sum  Inputs=+-
  Bus Creator : BusCreator  Inputs=3
  Bus Selector : BusSelector  OutputSignals=phi,mu
  Bus Selector1 : BusSelector  OutputSignals=value,derivative
  Bus Selector2 : BusSelector  OutputSignals=value,derivative
  Constant : Constant  Value=0.0
  If : If  NumInputs=2  IfExpression=u1 >= u2  ShowElse=off
  Product : Product  Inputs=3
  Product1 : Product
  initial_objective_function : Subsystem
  objective_function : Subsystem  TreatAsAtomicUnit=on
  f_u : Outport
  wires:
  psi/1 -> Bus Selector/1
  a_u/1 -> Bus Creator/1, objective_function/1(step_size), Product/2, If/1  "a_t"
  If/1 -> objective_function/Action
  Constant/1 -> initial_objective_function/1(step_size), If/2
  Bus Selector/1 -> initial_objective_function/2(phi), objective_function/2(phi)  "<phi>"
  localizer_ptr/1 -> initial_objective_function/3(localizer_ptr), objective_function/3(localizer_ptr)
  Product/1 -> Add/3
  Bus Selector/2 -> Product1/1, Product/1  "<mu>"
  objective_function/1(objective_function_value) -> Bus Selector1/1
  Bus Selector1/1 -> Add/1  "<value>"
  initial_objective_function/1(initial_objective_function_value) -> Bus Selector2/1
  Bus Selector2/1 -> Add/2  "<value>"
  Bus Selector2/2 -> Product1/2, Product/3  "<derivative>"
  Add/1 -> Bus Creator/2  "value"
  Bus Selector1/2 -> Add1/1  "<derivative>"
  Product1/1 -> Add1/2
  Add1/1 -> Bus Creator/3  "derivative"
  Bus Creator/1 -> f_u/1

== system NDT_Localization/observation_callback/check_localizer/If Action Subsystem/register_measurement_impl/If Action Subsystem/If Action Subsystem/solve/If Action Subsystem1/For Iterator Subsystem/compute_next_step/If Action Subsystem1/phi_0 ==
  step_size : Inport
  phi : Inport  Port=2
  localizer_ptr : Inport  Port=3
  Add : Sum
  Add4 : Sum  Inputs=+
  Bus Creator : BusCreator  Inputs=3
  Bus Selector : BusSelector  OutputSignals=eig_pose,opt_direction,problem
  Bus Selector1 : BusSelector  OutputSignals=scan,map
  Bus Selector2 : BusSelector  OutputSignals=vx.centroid,vx.inv_covariance
  Bus Selector3 : BusSelector  OutputSignals=outlier_ratio,localizer_config.map_config.voxel_size.x,localizer_config.map_config.voxel_size.y,localizer_config.map_config.voxel_size.z
  For Iterator Subsystem : Subsystem  TreatAsAtomicUnit=on
  Math Function2 : Math  Operator=square
  Product : Product
  Product{1..9} (9 alike) : Product  Multiplication=Matrix(*)
  angle_params : Subsystem
  gradient_angle : Subsystem
  point_gradient : MATLAB Function  TreatAsAtomicUnit=on
  set_jacobian : MATLAB Function  TreatAsAtomicUnit=on
  phi_0 : Outport
  wires:
  angle_params/1(params) -> gradient_angle/1(params)
  Bus Selector3/1 -> For Iterator Subsystem/4(outlier_ratio)  "<outlier_ratio>"
  gradient_angle/3(ga_c_out) -> Product4/2
  gradient_angle/4(ga_d_out) -> Product5/2
  gradient_angle/1(ga_a_out) -> Product2/2
  gradient_angle/6(ga_f_out) -> Product7/2
  Bus Selector2/2 -> For Iterator Subsystem/3(sigma)  "<inv_covariance>"
  Product5/1 -> point_gradient/4(ga_d)
  Product3/1 -> point_gradient/2(ga_b)
  set_jacobian/1(jacobian) -> For Iterator Subsystem/8(set_jacobian)
  Bus Selector1/1 -> Product9/1, Product8/1, Product7/1, Product6/1, Product5/1, Product4/1, Product3/1, Product2/1, For Iterator Subsystem/1(data)  "<scan>"
  Bus Selector/1 -> Add/1  "<eig_pose>"
  gradient_angle/7(ga_g_out) -> Product8/2
  Product8/1 -> point_gradient/7(ga_g)
  gradient_angle/8(ga_h_out) -> Product9/2
  Math Function2/1 -> Add4/1
  Product6/1 -> point_gradient/5(ga_e)
  Bus Selector2/1 -> For Iterator Subsystem/2(myu)  "<centroid>"
  localizer_ptr/1 -> Bus Selector3/1
  gradient_angle/5(ga_e_out) -> Product6/2
  gradient_angle/2(ga_b_out) -> Product3/2
  Add/1 -> Product/1
  Bus Selector/3 -> Bus Selector1/1  "<problem>"
  Product7/1 -> point_gradient/6(ga_f)
  Product9/1 -> point_gradient/8(ga_h)
  For Iterator Subsystem/2(jacobian_out) -> Product1/1
  Product/1 -> angle_params/1(pose)  "current_state"
  Add4/1 -> Product1/2, Product/2  "step_direction"
  Product2/1 -> point_gradient/1(ga_a)
  Bus Selector/2 -> Math Function2/1  "<opt_direction>"
  Bus Creator/1 -> phi_0/1
  Bus Selector1/2 -> Bus Selector2/1  "<map>"
  point_gradient/1(hessian) -> For Iterator Subsystem/9(set_gradient)
  Bus Selector3/3 -> For Iterator Subsystem/6(voxel_size_y)  "<y>"
  Bus Selector3/4 -> For Iterator Subsystem/7(voxel_size_z)  "<z>"
  phi/1 -> Bus Selector/1
  Bus Selector3/2 -> For Iterator Subsystem/5(voxel_size_x)  "<x>"
  Product4/1 -> point_gradient/3(ga_c)
  step_size/1 -> Bus Creator/1, Add/2  "step_size"
  For Iterator Subsystem/1(score_out) -> Bus Creator/2  "value"
  Product1/1 -> Bus Creator/3  "derivative"

== system NDT_Localization/observation_callback/check_localizer/If Action Subsystem/register_measurement_impl/If Action Subsystem/If Action Subsystem/solve/If Action Subsystem1/For Iterator Subsystem/compute_next_step/If Action Subsystem1/phi_t ==
  a_t : Inport
  phi : Inport  Port=2
  localizer_ptr : Inport  Port=3
  Action Port : ActionPort  ActionPortLabel=if(u1 >= u2)
  Add : Sum
  Add4 : Sum  Inputs=+
  Bus Creator : BusCreator  Inputs=3
  Bus Selector : BusSelector  OutputSignals=eig_pose,opt_direction,problem
  Bus Selector1 : BusSelector  OutputSignals=scan,map
  Bus Selector2 : BusSelector  OutputSignals=vx.centroid,vx.inv_covariance
  Bus Selector3 : BusSelector  OutputSignals=outlier_ratio,localizer_config.map_config.voxel_size.x,localizer_config.map_config.voxel_size.y,localizer_config.map_config.voxel_size.z
  For Iterator Subsystem : Subsystem  TreatAsAtomicUnit=on
  Math Function2 : Math  Operator=square
  Product : Product
  Product{1..9} (9 alike) : Product  Multiplication=Matrix(*)
  angle_params : Subsystem
  gradient_angle : Subsystem
  point_gradient : MATLAB Function  TreatAsAtomicUnit=on
  set_jacobian : MATLAB Function  TreatAsAtomicUnit=on
  phi_t : Outport
  wires:
  Add/1 -> Product/1
  a_t/1 -> Bus Creator/1, Add/2  "step_size"
  Product/1 -> angle_params/1(pose)  "current_state"
  Bus Selector/1 -> Add/1  "<eig_pose>"
  Add4/1 -> Product1/2, Product/2  "step_direction"
  phi/1 -> Bus Selector/1
  Bus Selector/2 -> Math Function2/1  "<opt_direction>"
  Math Function2/1 -> Add4/1
  Bus Selector/3 -> Bus Selector1/1  "<problem>"
  For Iterator Subsystem/2(jacobian_out) -> Product1/1
  Product1/1 -> Bus Creator/3  "derivative"
  Product9/1 -> point_gradient/8(ga_h)
  Product8/1 -> point_gradient/7(ga_g)
  Bus Selector2/2 -> For Iterator Subsystem/3(sigma)  "<inv_covariance>"
  gradient_angle/4(ga_d_out) -> Product5/2
  Product7/1 -> point_gradient/6(ga_f)
  Product6/1 -> point_gradient/5(ga_e)
  gradient_angle/6(ga_f_out) -> Product7/2
  Bus Selector1/1 -> Product9/1, Product8/1, Product7/1, Product6/1, Product5/1, Product4/1, Product3/1, Product2/1, For Iterator Subsystem/1(data)  "<scan>"
  point_gradient/1(hessian) -> For Iterator Subsystem/9(set_gradient)
  gradient_angle/2(ga_b_out) -> Product3/2
  gradient_angle/3(ga_c_out) -> Product4/2
  gradient_angle/7(ga_g_out) -> Product8/2
  gradient_angle/5(ga_e_out) -> Product6/2
  gradient_angle/8(ga_h_out) -> Product9/2
  Product5/1 -> point_gradient/4(ga_d)
  Product3/1 -> point_gradient/2(ga_b)
  Product4/1 -> point_gradient/3(ga_c)
  angle_params/1(params) -> gradient_angle/1(params)
  set_jacobian/1(jacobian) -> For Iterator Subsystem/8(set_jacobian)
  Bus Selector1/2 -> Bus Selector2/1  "<map>"
  gradient_angle/1(ga_a_out) -> Product2/2
  Product2/1 -> point_gradient/1(ga_a)
  Bus Selector2/1 -> For Iterator Subsystem/2(myu)  "<centroid>"
  localizer_ptr/1 -> Bus Selector3/1
  Bus Selector3/1 -> For Iterator Subsystem/4(outlier_ratio)  "<outlier_ratio>"
  Bus Selector3/2 -> For Iterator Subsystem/5(voxel_size_x)  "<x>"
  Bus Selector3/3 -> For Iterator Subsystem/6(voxel_size_y)  "<y>"
  Bus Selector3/4 -> For Iterator Subsystem/7(voxel_size_z)  "<z>"
  For Iterator Subsystem/1(score_out) -> Bus Creator/2  "value"
  Bus Creator/1 -> phi_t/1
